simulink model "gm_compar"  (R2024b)
settings: Solver=FixedStepDiscrete  StartTime=0.0  StopTime=10.0  RelTol=1e-3
settings Model: Creator=Angel  LastModifiedBy=Angel
settings OptimizationCC: BlockReduction=off  ConditionallyExecuteInputs=off  DefaultParameterBehavior=Inlined
settings DebuggingCC: AlgebraicLoopMsg=error  InheritedTsInSrcMsg=none
settings HardwareCC: ProdBitPerPointer=32  ProdBitPerSizeT=32  ProdBitPerPtrDiffT=32  ProdLargestAtomicFloat=None  ProdIntDivRoundTo=Undefined  ProdEndianess=Unspecified  ProdWordSize=32  ProdHWDeviceType=ASIC/FPGA->ASIC/FPGA  TargetBitPerPointer=64  TargetBitPerSizeT=64  TargetBitPerPtrDiffT=64  TargetLongLongMode=on  TargetIntDivRoundTo=Zero  TargetEndianess=LittleEndian  TargetWordSize=64  TargetHWDeviceType=Custom Processor->MATLAB Host Computer  ProdEqTarget=off

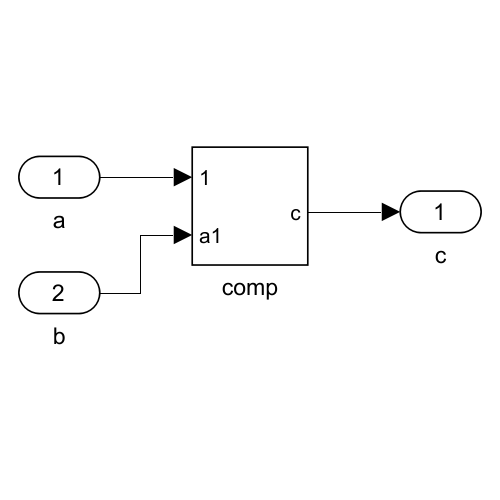
[thumbnail: Simulink's stored preview of the top-level diagram]
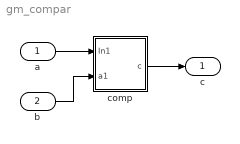
== system gm_compar ==
  a : Inport  OutDataTypeStr=uint16  PortDimensions=1  SampleTime=0.2
  b : Inport  Port=2  OutDataTypeStr=uint16  PortDimensions=1  SampleTime=0.2
  comp : Subsystem
  c : Outport  SampleTime=0.2
  wires:
  a/1 -> comp/1(In1)
  b/1 -> comp/2(a1)
  comp/1(c) -> c/1

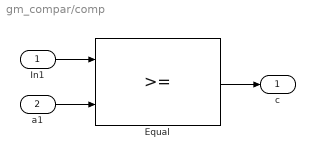
== system gm_compar/comp ==
  In1 : Inport  OutDataTypeStr=uint16  PortDimensions=1  SampleTime=0.2
  a1 : Inport  Port=2  OutDataTypeStr=uint16  PortDimensions=1  SampleTime=0.2
  Equal : RelationalOperator  OutDataTypeStr=boolean  ZeroCross=off  RndMeth=Floor  InputSameDT=off
  c : Outport  SampleTime=0.2
  wires:
  In1/1 -> Equal/1
  a1/1 -> Equal/2
  Equal/1 -> c/1
